simulink model "DT_NL_TORA"  (R2019b)
settings: Solver=FixedStepDiscrete  StartTime=0.0  StopTime=stoptime  FixedStep=Ts  MaxStep=Ts  RelTol=1e-6  AbsTol=1e-6
values from neighbouring files (symbols this model uses):
  Ad = matexp(A,Ts,n)    [mainfile_solution.m]
  Bd = intmatexpB(A,B,Ts,n)    [mainfile_solution.m]
  Cd = sysdzoh.C    [mainfile_solution.m]
  Dd = sysdzoh.D    [mainfile_solution.m]
  Kd = place(Ad,Bd,p_z)    [mainfile_solution.m]
  Ts = 0.01    [mainfile_solution.m]
  x0 = [20*pi/180 , 0 ,  0.1 , 0]'    [mainfile_solution.m]
  x_bar = [0 0 0 0]'    [mainfile_solution.m]
settings Model: Creator=Ale  LastModifiedBy=don
settings SolverCC: AutoScaleAbsTol=off
settings DataIOCC: SaveFormat=Array  SignalLoggingSaveFormat=ModelDataLogs  SaveOutput=off  SaveTime=off  TimeSaveName=t
settings OptimizationCC: ExpressionDepthLimit=2147483647  LifeSpan=inf
settings DebuggingCC: UnderspecifiedInitializationDetection=Classic  MergeDetectMultiDrivingBlocksExec=none  FcnCallInpInsideContextMsg=warning  StateNameClashWarn=warning  SFUnexpectedBacktrackingDiag=warning  SFNoUnconditionalDefaultTransitionDiag=warning  SFExecutionAtInitializationDiag=none  ArithmeticOperatorsInVariantConditions=warning
settings HardwareCC: ProdBitPerPointer=32  ProdBitPerSizeT=32  ProdBitPerPtrDiffT=32  ProdLargestAtomicFloat=None  ProdIntDivRoundTo=Undefined  ProdEndianess=Unspecified  ProdWordSize=32  ProdHWDeviceType=32-bit Generic
settings ModelReferenceCC: PropagateSignalLabelsOutOfModel=off
settings SFSimCC: SimUseLocalCustomCode=off  CustomCodeUndefinedFunction=UseInterfaceOnly
settings RTWCC: RTWUseLocalCustomCode=off
settings CodeAppCC: StateflowObjectComments=on
settings GRTTargetCC: TargetLangStandard=C89/C90 (ANSI)  GeneratePreprocessorConditionals=Disable all  CombineOutputUpdateFcns=off  GRTInterface=on
settings ConfigComp: CovMetricSettings=dw  CovHtmlReporting=on  CovSaveCumulativeToWorkspaceVar=on  CovSaveSingleToWorkspaceVar=on  CovExternalEMLEnable=off

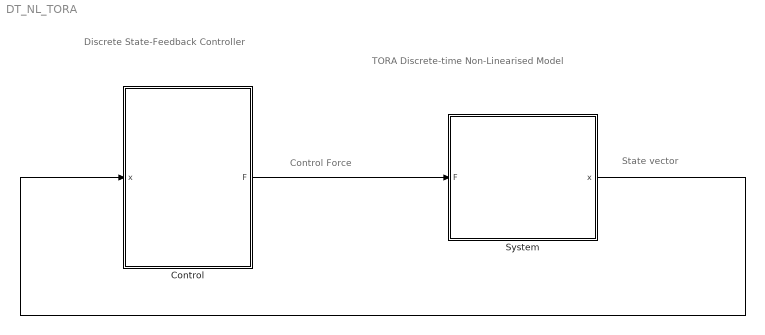
== system DT_NL_TORA ==
  note: Discrete State-Feedback
      | Controller
  note: Control Force
  note: State vector
  note: TORA
      | Discrete-time Non-Linearised Model
  Control : Subsystem
  System : Subsystem
  wires:
  System/1(x) -> Control/1(x)
  Control/1(F) -> System/1(F)

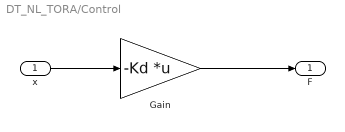
== system DT_NL_TORA/Control ==
  x : Inport
  Gain : Gain  Gain=-Kd  Multiplication=Matrix(K*u)
  F : Outport  VectorParamsAs1DForOutWhenUnconnected=off
  wires:
  x/1 -> Gain/1
  Gain/1 -> F/1

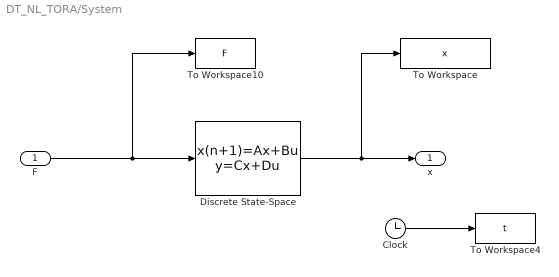
== system DT_NL_TORA/System ==
  F : Inport
  Clock : Clock
  Discrete State-Space : DiscreteStateSpace  A=Ad  B=Bd  C=Cd  D=Dd  InitialCondition=x0 - x_bar  SampleTime=Ts
  To Workspace : ToWorkspace  VariableName=x  SampleTime=Ts
  To Workspace10 : ToWorkspace  VariableName=F  SampleTime=Ts
  To Workspace4 : ToWorkspace  VariableName=t  SampleTime=Ts
  x : Outport  VectorParamsAs1DForOutWhenUnconnected=off
  wires:
  F/1 -> Discrete State-Space/1, To Workspace10/1
  Discrete State-Space/1 -> To Workspace/1, x/1
  Clock/1 -> To Workspace4/1
